simulink model "Glider6"  (R2019a)
settings: Solver=ode4  StartTime=0.0  StopTime=200  FixedStep=0.1  RelTol=1e-3
libraries: simulink x1
settings Model: Creator=whsteyn  LastModifiedBy=Wian
settings SolverCC: AlgebraicLoopSolver=LineSearch
settings DataIOCC: LimitDataPoints=on  SaveFormat=Array  ReturnWorkspaceOutputs=off
settings OptimizationCC: InitFltsAndDblsToZero=on  LifeSpan=inf
settings DebuggingCC: SaveWithParameterizedLinksMsg=none  UnderspecifiedInitializationDetection=Classic  MergeDetectMultiDrivingBlocksExec=none  SignalResolutionControl=TryResolveAllWithWarning  SolverPrmCheckMsg=warning  MultiTaskDSMMsg=warning  MultiTaskCondExecSysMsg=none  FcnCallInpInsideContextMsg=warning  SFUnexpectedBacktrackingDiag=warning  SFNoUnconditionalDefaultTransitionDiag=warning  SFExecutionAtInitializationDiag=none  ArithmeticOperatorsInVariantConditions=warning
settings HardwareCC: ProdBitPerPointer=32  ProdBitPerSizeT=32  ProdBitPerPtrDiffT=32  ProdLargestAtomicFloat=None  ProdIntDivRoundTo=Undefined  ProdEndianess=Unspecified  ProdWordSize=32  ProdHWDeviceType=32-bit Generic
settings ModelReferenceCC: PropagateSignalLabelsOutOfModel=off
settings SFSimCC: SimUseLocalCustomCode=off
settings RTWCC: RTWUseLocalCustomCode=off
settings CodeAppCC: StateflowObjectComments=on
settings GRTTargetCC: TargetFcnLib=ansi_tfl_tmw.mat  TargetLangStandard=C89/C90 (ANSI)  GeneratePreprocessorConditionals=Disable all  CombineOutputUpdateFcns=off  GRTInterface=on
settings ConfigComp: CovMetricSettings=dw  CovHtmlReporting=on  CovSaveCumulativeToWorkspaceVar=on  CovSaveSingleToWorkspaceVar=on  CovExternalEMLEnable=off  CovSFcnEnable=off

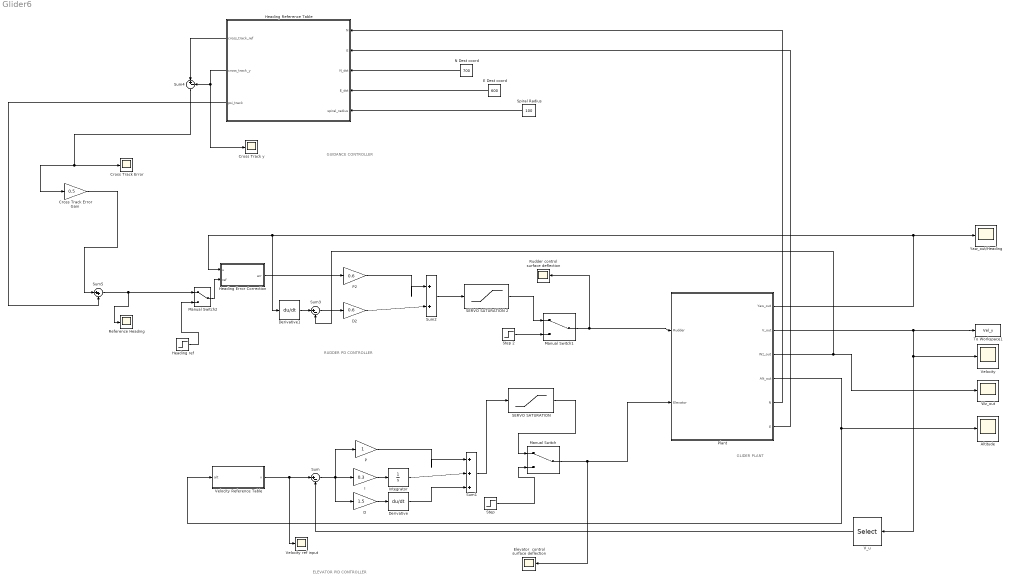
== system Glider6 ==
  note: GLIDER PLANT
  note: RUDDER PD CONTROLLER
  note: ELEVATOR PID CONTROLLER
  note: GUIDANCE CONTROLLER
  Altitude : Scope
  Cross Track Error : Scope
  Cross Track Error Gain : Gain  Gain=0.5
  Cross Track y : Scope
  D : Gain  Gain=1.5
  D2 : Gain  Gain=0.6
  Derivative : Derivative
  Derivative1 : Derivative
  E Dest coord : Constant  Value=600
  Elevator  control surface deflection : Scope
  Heading Error Correction : MATLAB Function  TreatAsAtomicUnit=on
  Heading Reference Table : MATLAB Function  TreatAsAtomicUnit=on
  Heading ref : Step  Time=20  After=160  SampleTime=0
  I : Gain  Gain=0.3
  Integrator : Integrator
  Manual Switch : ManualSwitch
  Manual Switch1 : ManualSwitch
  Manual Switch2 : ManualSwitch
  N Dest coord : Constant  Value=700
  P : Gain
  P2 : Gain  Gain=0.6
  Plant : Subsystem
  Reference Heading : Scope
  Rudder control surface deflection : Scope
  SERVO SATURATION : Saturate  UpperLimit=10  LowerLimit=-10
  SERVO SATURATION 2 : Saturate  UpperLimit=10  LowerLimit=-10  LinearizeAsGain=off
  Spiral Radius : Constant  Value=100
  Step : Step  After=0.05  SampleTime=0
  Step 2 : Step  After=0.1  SampleTime=0
  Sum : Sum  Inputs=|+-
  Sum1 : Sum  Inputs=|+++
  Sum2 : Sum  Inputs=|++
  Sum3 : Sum  Inputs=|+-
  Sum4 : Sum  Inputs=|+-
  Sum5 : Sum  Inputs=|++
  To Workspace1 : ToWorkspace  VariableName=Vel_y  SampleTime=-1
  V_u : Selector  InputPortWidth=3  IndexOptions=Index vector (dialog)  Indices=[1]  OutputSizes=1
  Velocity : Scope
  Velocity Reference Table : MATLAB Function  TreatAsAtomicUnit=on
  Velocity ref input : Scope
  Wz_out : Scope
  "Yaw_out/Heading " : Scope
  wires:
  D/1 -> Derivative/1
  I/1 -> Integrator/1
  Sum/1 -> P/1, D/1, I/1
  P/1 -> Sum1/1
  Integrator/1 -> Sum1/2
  Derivative/1 -> Sum1/3
  Sum1/1 -> SERVO SATURATION/1
  Velocity Reference Table/1(v) -> Sum/1, Velocity ref input/1
  Plant/4(Alt_out) -> Altitude/1, Velocity Reference Table/1(alt)
  Manual Switch/1 -> Plant/2(Elevator), Elevator  control surface deflection/1
  SERVO SATURATION/1 -> Manual Switch/1
  Step/1 -> Manual Switch/2
  Step 2/1 -> Manual Switch1/2
  Manual Switch1/1 -> Rudder control surface deflection/1, Plant/1(Rudder)
  SERVO SATURATION 2/1 -> Manual Switch1/1
  Sum2/1 -> SERVO SATURATION 2/1
  P2/1 -> Sum2/1
  Plant/1(Yaw_out) -> "Yaw_out/Heading "/1, Derivative1/1, Heading Error Correction/1(u)
  Plant/2(V_out) -> To Workspace1/1, V_u/1, Velocity/1
  V_u/1 -> Sum/2
  Plant/3(Wz_out) -> Sum3/2, Wz_out/1
  Sum3/1 -> D2/1
  Heading Error Correction/1(err) -> P2/1
  D2/1 -> Sum2/2
  Derivative1/1 -> Sum3/1
  Plant/5(N) -> Heading Reference Table/1(N)
  Plant/6(E) -> Heading Reference Table/2(E)
  Heading Reference Table/1(cross_track_ref) -> Sum4/1
  Sum4/1 -> Cross Track Error Gain/1, Cross Track Error/1
  Cross Track Error Gain/1 -> Sum5/1
  Sum5/1 -> Manual Switch2/1, Reference Heading/1
  Heading Reference Table/2(cross_track_y) -> Cross Track y/1, Sum4/2
  Heading Reference Table/3(psi_track) -> Sum5/2
  N Dest coord/1 -> Heading Reference Table/3(N_dst)
  E Dest coord/1 -> Heading Reference Table/4(E_dst)
  Heading ref/1 -> Manual Switch2/2
  Manual Switch2/1 -> Heading Error Correction/2(ref)
  Spiral Radius/1 -> Heading Reference Table/5(spiral_radius)

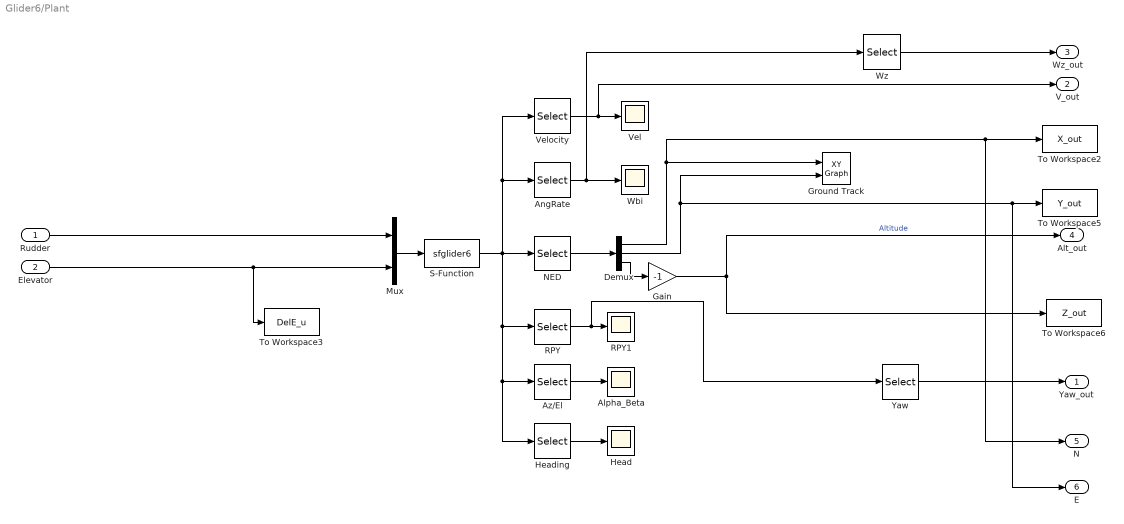
== system Glider6/Plant ==
  Rudder : Inport
  Elevator : Inport  Port=2
  Alpha_Beta : Scope
  AngRate : Selector  InputPortWidth=15  IndexOptions=Index vector (dialog)  Indices=[4:6]  OutputSizes=1
  Az/El : Selector  InputPortWidth=15  IndexOptions=Index vector (dialog)  Indices=[13,14]  OutputSizes=1
  Demux : Demux  Outputs=3
  Gain : Gain  Gain=-1
  Ground Track : simulink/Sinks/XY Graph  xmin=-1000  xmax=3000  ymin=-1000  ymax=1000  st=-1
  Head : Scope
  Heading : Selector  InputPortWidth=15  IndexOptions=Index vector (dialog)  Indices=[13,14]  OutputSizes=1
  Mux : Mux  Inputs=2
  NED : Selector  InputPortWidth=15  IndexOptions=Index vector (dialog)  Indices=[7:9]  OutputSizes=1
  RPY : Selector  InputPortWidth=15  IndexOptions=Index vector (dialog)  Indices=[10:12]  OutputSizes=1
  RPY1 : Scope
  S-Function : S-Function  FunctionName=sfglider6  Parameters=2100,2.5,[12.2 0 0.8],[0 -4 0]  SFunctionDeploymentMode=off  EnableBusSupport=off
  To Workspace2 : ToWorkspace  VariableName=X_out  SampleTime=-1
  To Workspace3 : ToWorkspace  VariableName=DelE_u  SampleTime=-1
  To Workspace5 : ToWorkspace  VariableName=Y_out  SampleTime=-1
  To Workspace6 : ToWorkspace  VariableName=Z_out  SampleTime=-1
  Vel : Scope
  Velocity : Selector  InputPortWidth=15  IndexOptions=Index vector (dialog)  Indices=[1:3]  OutputSizes=1
  Wbi : Scope
  Wz : Selector  InputPortWidth=3  IndexOptions=Index vector (dialog)  Indices=[3]  OutputSizes=1
  Yaw : Selector  InputPortWidth=3  IndexOptions=Index vector (dialog)  Indices=[3]  OutputSizes=1
  Yaw_out : Outport
  V_out : Outport  Port=2
  Wz_out : Outport  Port=3
  Alt_out : Outport  Port=4
  N : Outport  Port=5
  E : Outport  Port=6
  wires:
  RPY/1 -> Yaw/1, RPY1/1
  Mux/1 -> S-Function/1
  Velocity/1 -> V_out/1, Vel/1
  Az/El/1 -> Alpha_Beta/1
  Demux/2 -> Ground Track/2, E/1, To Workspace5/1
  Demux/1 -> N/1, To Workspace2/1, Ground Track/1
  S-Function/1 -> AngRate/1, Velocity/1, NED/1, RPY/1, Heading/1, Az/El/1
  Heading/1 -> Head/1
  NED/1 -> Demux/1
  Gain/1 -> Alt_out/1, To Workspace6/1  "Altitude"
  Rudder/1 -> Mux/1
  AngRate/1 -> Wbi/1, Wz/1
  Demux/3 -> Gain/1
  Elevator/1 -> To Workspace3/1, Mux/2
  Yaw/1 -> Yaw_out/1
  Wz/1 -> Wz_out/1

== matlab function Glider6/Velocity Reference Table ==
  data: alt input; v output
% Change velocity reference as a function of altitude
function v = fcn(alt)

if alt < 1000
   v = 10.97;
   
elseif alt >= 1000 && alt < 2000
   v = 11.25;
   
elseif alt > 2000 && alt < 3000
   v = 11.8;
  
elseif alt > 3000 && alt < 4000
   v = 12.5;
   
elseif alt > 4000 && alt < 5000
   v = 13.4;
   
elseif alt > 5000 && alt < 6000
   v = 14.5;
   
elseif alt > 6000 && alt < 7000
   v = 16.0;
   
elseif alt > 7000 && alt < 8000
   v = 18.0;
   
elseif alt > 8000 && alt < 9000
   v = 21.0;
   
elseif alt > 9000 && alt < 10000
   v = 26.2;
   
else
    v = 38.2;
end   



end

== matlab function Glider6/Heading Reference Table ==
  data: cross_track_ref output; cross_track_y output; N input; E input; psi_track output; N_dst input; E_dst input; spiral_radius input
% Calculate Heading Reference Input
function  [cross_track_ref,cross_track_y, psi_track] = fcn(N,E,N_dst,E_dst, spiral_radius)

% Balloon Release Coordinate 
N_src = 0;
E_src = 0;

% Radius between aircraft and airport center point
R = sqrt((N-N_dst).^2 + (E-E_dst).^2);

 if R < spiral_radius + 100
    % Calculate psi_track error for current orientation
    psi_track = atan2((E-E_dst),(N-N_dst))*180/pi;
    if psi_track < 0
       psi_track = 360 + psi_track;
    end
    psi_track = psi_track - 90;
    cross_track_y = sqrt((N-N_dst).^2 + (E-E_dst).^2);
    cross_track_ref = spiral_radius;
    % If outside circle
    if cross_track_y > cross_track_ref
    cross_track_y = sqrt((N-N_dst).^2 + (E-E_dst).^2);
    % If inside circle
    elseif cross_track_y < cross_track_ref
    cross_track_y = -sqrt((N-N_dst).^2 + (E-E_dst).^2);
    end
    
 else
 
 % Fly to airport from balloon release point
 cross_track_ref = 0;
 psi_track = atan2((E_dst-E_src),(N_dst-N_src))*180/pi;
    if psi_track < 0
       psi_track = 360 + psi_track;
    end
 cross_track_y = -sin(psi_track*pi/180)*(N-N_src) + cos(psi_track*pi/180)*(E-E_src);
 
end


end

== matlab function Glider6/Heading Error Correction ==
  data: err output; u input; ref input
% Correct Heading error from reference input and determine shortest yaw
% turn angle
% Input angles u must be normalised to +/-180 degrees axis system
% - error = Turn Left
% + error = Turn Right
function err = heading_err(u,ref)

% Normalise reference to +/-180 degrees axis system
if ref > 180
ref = ref - 360;
else 
end

% Calculate shortest turn angle error 
turn = ref - u;

if turn > 180
err = -(turn - 360);
%err = -t;
elseif turn < -180
err = (abs(turn) - 360);
%err = -t;
else
err = -turn;
end


end
